simulink library "PELIIONPACK01MSEREF"  (R2014b)
settings: Solver=ode45  StartTime=0.0  StopTime=10.0  RelTol=1e-3
undefined symbols (not defined in the file): errordlg
libraries: simulink x19
settings Model: Creator=NMN6KOR  LastModifiedBy=hj82sh

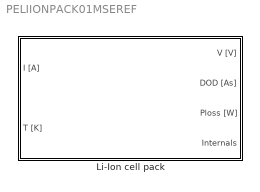
== system PELIIONPACK01MSEREF ==
  Li-Ion cell pack : Subsystem  Tag=PELIIONPACK01MSEREF  mask(PELIIONPACK01MSEREF){NumCell=1, DODtab=[0 : 23.5176 : 4680 4680], Ttab=[250 261 272 283 294 305 316 327 338 350], Vocvtab=|, Rhf=35e-3, Csn=0.01, Rct=40e-3, Cdl=700, rho=0.5, I0=0.5, T0=1.4e3, D_Rhf=[1], D_Rct=[1], D_ocv=[1], DODinit=0, VRhfinit=0, Vdlinit=0}
      mask Vocvtab=|
      | repmat( [4.10 4.09 4.09 4.08 4.08 4.08 4.08 4.07 4.07 4.07, ...
      |  4.07 4.06 4.06 4.06 4.06 4.06 4.05 4.05 4.05 4.05, ...
      |  4.05 4.04 4.04 4.04 4.04 4.04 4.03 4.03 4.03 4.02, ...
      |  4.02 4.02 4.01 4.01 4.01 4.00 4.00 3.99 3.99 3.99, ...
      |  3.98 3.98 3.98 3.97 3.97 3.96 3.96 3.96 3.95 3.95, ...
      |  3.95 3.94 3.94 3.94 3.94 3.93 3.93 3.93 3.92 3.92, ...
      |  3.92 3.92 3.91 3.91 3.91 3.90 3.90 3.90 3.89 3.89, ...
      |  3.88 3.88 3.87 3.87 3.86 3.86 3.86 3.86 3.85 3.85, ...
      |  3.85 3.84 3.84 3.84 3.84 3.83 3.83 3.83 3.82 3.82, ...
      |  3.82 3.81 3.81 3.81 3.80 3.80 3.80 3.79 3.79 3.78, ...
      |  3.78 3.78 3.77 3.77 3.76 3.76 3.75 3.75 3.74 3.74, ...
      |  3.73 3.73 3.72 3.72 3.71 3.71 3.70 3.70 3.69 3.69, ...
      |  3.68 3.68 3.67 3.67 3.67 3.66 3.66 3.65 3.65 3.65, ...
      |  3.64 3.64 3.63 3.63 3.63 3.62 3.62 3.62 3.61 3.61, ...
      |  3.60 3.60 3.60 3.59 3.59 3.58 3.58 3.58 3.57 3.57, ...
      |  3.56 3.56 3.55 3.55 3.54 3.54 3.53 3.53 3.52 3.51, ...
      |  3.51 3.50 3.50 3.49 3.48 3.48 3.47 3.47 3.46 3.45, ...
      |  3.45 3.44 3.43 3.43 3.42 3.42 3.41 3.41 3.40 3.40, ...
      |  3.39 3.39 3.38 3.37 3.37 3.36 3.35 3.34 3.33 3.31, ...
      |  3.29 3.26 3.23 3.20 3.17 3.12 3.07 3.00 2.91 2.76]', 1, 10 )
      mask prompts: NumCell "Number of cells in series connection"; DODtab "Vocv table DOD-axis [As]"; Ttab "Vocv table T-axis [K]"; Vocvtab "Vocv table [V]"; Rhf "High frequency resistance [Ohm]"; Csn "Snubber capacitance [F]"; Rct "Charge transfer resistance [Ohm]"; Cdl "Double layer capacitance [F]"; rho "Weighting factor for current dependency [-]"; I0 "Scale factor for current dependency [A]"; T0 "Scale factor for temperature dependency [K]"; D_Rhf "Rhf deviation vector [-]"; D_Rct "Rct deviation vector [-]"; D_ocv "Vocv deviation vector [-]"; DODinit "Initial depth of discharge [As]"; VRhfinit "Initial high frequency resistor voltage [V]"; Vdlinit "Initial double layer voltage [V]"
      mask help:
      | PELIIONPACK01MSEREF - Li-Ion cell pack model
      |
      | This is a simple equivalent circuit model for a series connection of Li-Ion secondary batteries. This impedance model describes the dynamical behavior of arbitrarily many cells connected in series (a subcase of this is the model of the single Li-Ion cell).
      | The number of cells determines the dimension of the input temperature vector.
      settings: AttributesFormatString=<%<Tag>>
      mask Help: eval('show_docs_mseref_powerelectronics(''PELIIONPACK01MSEREF'')')
      mask Display:
      | image(imread('PELIIONPACK01MSEREF_icon.png'))
      | port_label('input',1,'I [A]')
      | port_label('input',2,'T [K]')
      | port_label('output',1,'V [V]')
      | port_label('output',2,'DOD [As]')
      | port_label('output',3,'Ploss [W]')
      | port_label('output',4,'Internals')

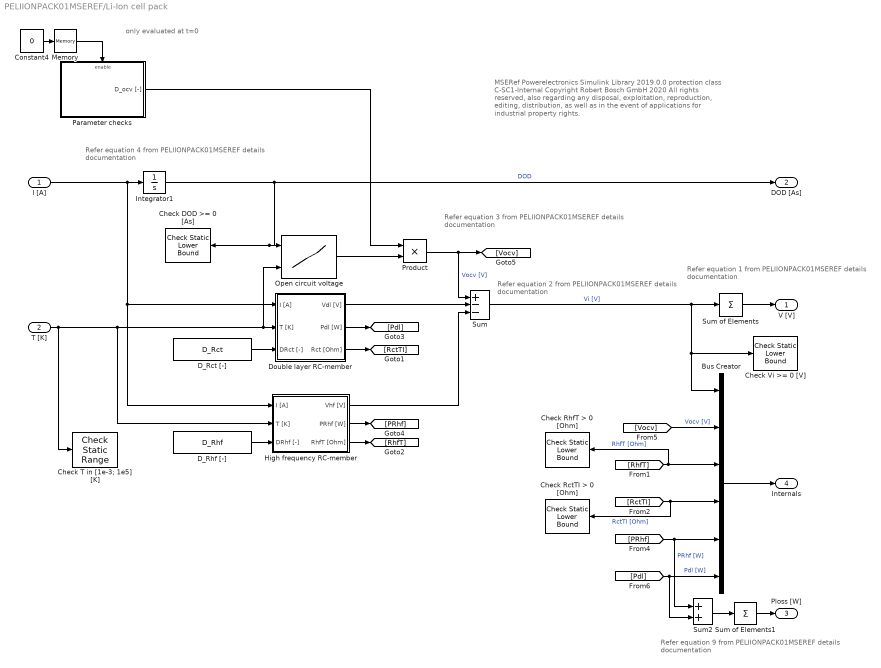
== system PELIIONPACK01MSEREF/Li-Ion cell pack ==
  note: Refer equation 9 from
      | PELIIONPACK01MSEREF details documentation
  note: Refer equation 2 from
      | PELIIONPACK01MSEREF details documentation
  note: Refer equation 4 from
      | PELIIONPACK01MSEREF details documentation
  note: only evaluated at t=0
  note: MSERef Powerelectronics Simulink Library 2019.0.0
      | protection class C-SC1-Internal
      |
      | Copyright Robert Bosch GmbH 2020
      |
      | All rights reserved, also regarding any disposal, exploitation,
      | reproduction, editing, distribution, as well as in the event of
      | applications for industrial property rights.
  note: Refer equation 1 from
      | PELIIONPACK01MSEREF details documentation
  note: Refer equation 3 from
      | PELIIONPACK01MSEREF details documentation
  I [A] : Inport
  T [K] : Inport  Port=2
  Bus Creator : BusCreator  Inputs=6
  Check DOD >= 0 [As] : simulink/Model Verification/Check Static  Lower Bound  Description=0 <= u  min=0  min_included=on  enabled=on  callback=errordlg('Output depth of discharge `DOD` has to be greater or equal to zero [As].')  stopWhenAssertionFail=on  export=off  icon=graphic
  Check RctTI > 0 [Ohm] : simulink/Model Verification/Check Static  Lower Bound  Description=0 <= u  min=0  min_included=on  enabled=on  callback=errordlg('Internal variable `RctTI` must have elements greater than zero [Ohm]. Possible reasons: Input port 3 `DeviVec`is unconnected, grounded or RhfT,i resp. RctTI,i is equal to zero.')  stopWhenAssertionFail=on  export=off  icon=graphic
  Check RhfT > 0 [Ohm] : simulink/Model Verification/Check Static  Lower Bound  Description=0 <= u  min=0  min_included=on  enabled=on  callback=errordlg('Internal variable `RhfT` must have elements greater than zero [Ohm]. Possible reasons: Input port 3 `DeviVec`is unconnected, grounded or RhfT,i resp. RctTI,i is equal to zero.')  stopWhenAssertionFail=on  export=off  icon=graphic
  Check Vi >= 0 [V] : simulink/Model Verification/Check Static  Lower Bound  Description=0 <= u  min=0  min_included=on  enabled=on  callback=errordlg('Terminal voltage `Vi` has to be greater or equal to zero [V].')  stopWhenAssertionFail=on  export=off  icon=graphic
  Check T in [1e-3; 1e5] [K] : simulink/Model Verification/Check  Static Range  Description=1e-3 <= u <= 1e5  max=1e5  max_included=on  min=1e-3  min_included=on  enabled=on  callback=errordlg('Input temperature `T` outside of range [1e-3; 1e5] [K].')  stopWhenAssertionFail=on  export=off  icon=graphic
  Constant4 : Constant  Value=0
  D_Rct [-] : Constant  Value=D_Rct
  D_Rhf [-] : Constant  Value=D_Rhf
  Double layer RC-member : Subsystem
  High frequency RC-member : Subsystem
  Integrator1 : Integrator  InitialCondition=DODinit
  Memory : Memory  X0=1
  Open circuit voltage : Lookup2D  RowIndex=DODtab  ColumnIndex=Ttab  Table=Vocvtab  LookUpMeth=Interpolation-Use End Values
  Parameter checks : Subsystem
  Product : Product
  Sum : Sum  Inputs=+--
  Sum of Elements : Sum  Inputs=+
  Sum of Elements1 : Sum  Inputs=+
  Sum2 : Sum
  V [V] : Outport
  DOD [As] : Outport  Port=2
  Ploss [W] : Outport  Port=3
  Internals : Outport  Port=4
  wires:
  Memory/1 -> Parameter checks/Enable
  Constant4/1 -> Memory/1
  Integrator1/1 -> Open circuit voltage/1, Check DOD >= 0 [As]/1, DOD [As]/1  "DOD"
  High frequency RC-member/3(RhfT [Ohm]) -> [RhfT]
  Double layer RC-member/3(Rct [Ohm]) -> [RctTI]
  Bus Creator/1 -> Internals/1
  High frequency RC-member/2(PRhf [W]) -> [PRhf]
  Double layer RC-member/2(Pdl [W]) -> [Pdl]
  T [K]/1 -> High frequency RC-member/2(T [K]), Double layer RC-member/2(T [K]), Open circuit voltage/2, Check T in [1e-3; 1e5] [K]/1
  Sum2/1 -> Sum of Elements1/1
  High frequency RC-member/1(Vhf [V]) -> Sum/3
  Double layer RC-member/1(Vdl [V]) -> Sum/2
  Open circuit voltage/1 -> Product/2
  I [A]/1 -> High frequency RC-member/1(I [A]), Double layer RC-member/1(I [A]), Integrator1/1
  [RhfT] -> Bus Creator/3, Check RhfT > 0 [Ohm]/1  "RhfT [Ohm]"
  [Vocv] -> Bus Creator/2  "Vocv [V]"
  Sum/1 -> Sum of Elements/1, Check Vi >= 0 [V]/1, Bus Creator/1  "Vi [V]"
  [RctTI] -> Check RctTI > 0 [Ohm]/1, Bus Creator/4  "RctTI [Ohm]"
  [PRhf] -> Sum2/1, Bus Creator/5  "PRhf [W]"
  [Pdl] -> Sum2/2, Bus Creator/6  "Pdl [W]"
  D_Rhf [-]/1 -> High frequency RC-member/3(DRhf [-])
  D_Rct [-]/1 -> Double layer RC-member/3(DRct [-])
  Sum of Elements/1 -> V [V]/1
  Product/1 -> Sum/1, [Vocv]  "Vocv [V]"
  Parameter checks/1(D_ocv [-]) -> Product/1
  Sum of Elements1/1 -> Ploss [W]/1

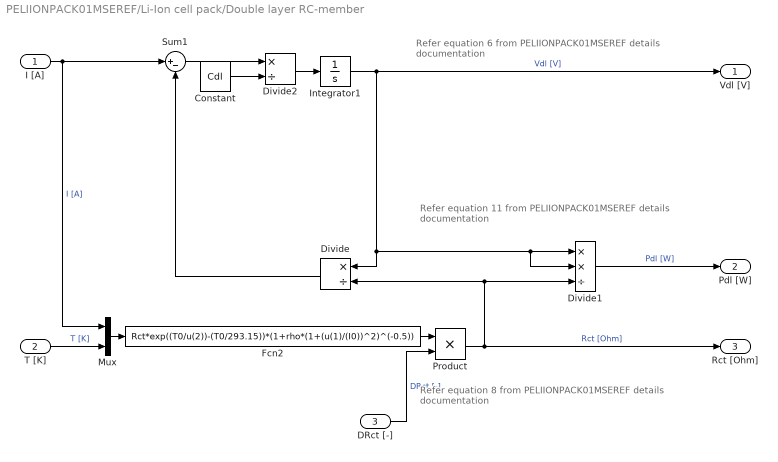
== system PELIIONPACK01MSEREF/Li-Ion cell pack/Double layer RC-member ==
  note: Refer equation 6 from
      | PELIIONPACK01MSEREF details documentation
  note: Refer equation 11 from
      | PELIIONPACK01MSEREF details documentation
  note: Refer equation 8 from
      | PELIIONPACK01MSEREF details documentation
  I [A] : Inport
  T [K] : Inport  Port=2
  DRct [-] : Inport  Port=3
  Constant : Constant  Value=Cdl
  Divide : Product  Inputs=*/
  Divide1 : Product  Inputs=**/
  Divide2 : Product  Inputs=*/
  Fcn2 : Fcn  Expr=Rct*exp((T0/u(2))-(T0/293.15))*(1+rho*(1+(u(1)/(I0))^2)^(-0.5))
  Integrator1 : Integrator  InitialCondition=Vdlinit
  Mux : Mux  Inputs=2
  Product : Product
  Sum1 : Sum  Inputs=|+-
  Vdl [V] : Outport
  Pdl [W] : Outport  Port=2
  Rct [Ohm] : Outport  Port=3
  wires:
  T [K]/1 -> Mux/2  "T [K]"
  Divide2/1 -> Integrator1/1
  Sum1/1 -> Divide2/1
  Divide1/1 -> Pdl [W]/1  "Pdl [W]"
  I [A]/1 -> Sum1/1, Mux/1  "I [A]"
  Product/1 -> Rct [Ohm]/1, Divide1/3, Divide/2  "Rct [Ohm]"
  Integrator1/1 -> Divide1/2, Divide1/1, Divide/1, Vdl [V]/1  "Vdl [V]"
  Divide/1 -> Sum1/2
  Constant/1 -> Divide2/2
  DRct [-]/1 -> Product/2  "DRct [-]"
  Mux/1 -> Fcn2/1
  Fcn2/1 -> Product/1

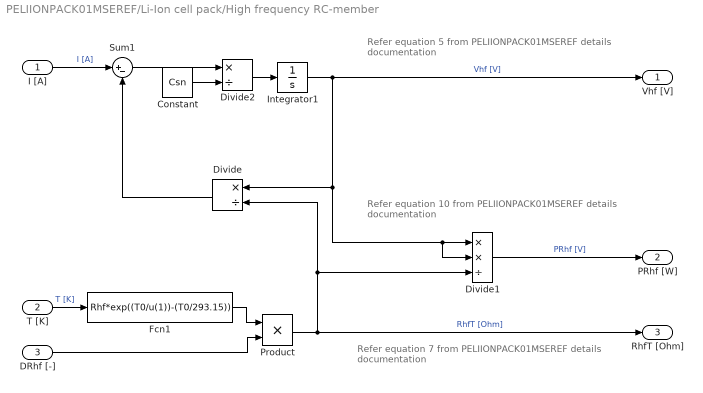
== system PELIIONPACK01MSEREF/Li-Ion cell pack/High frequency RC-member ==
  note: Refer equation 7 from
      | PELIIONPACK01MSEREF details documentation
  note: Refer equation 5 from
      | PELIIONPACK01MSEREF details documentation
  note: Refer equation 10 from
      | PELIIONPACK01MSEREF details documentation
  I [A] : Inport
  T [K] : Inport  Port=2
  DRhf [-] : Inport  Port=3
  Constant : Constant  Value=Csn
  Divide : Product  Inputs=*/
  Divide1 : Product  Inputs=**/
  Divide2 : Product  Inputs=*/
  Fcn1 : Fcn  Expr=Rhf*exp((T0/u(1))-(T0/293.15))
  Integrator1 : Integrator  InitialCondition=VRhfinit
  Product : Product
  Sum1 : Sum  Inputs=|+-
  Vhf [V] : Outport
  PRhf [W] : Outport  Port=2
  RhfT [Ohm] : Outport  Port=3
  wires:
  Divide1/1 -> PRhf [W]/1  "PRhf [V]"
  Divide2/1 -> Integrator1/1
  Divide/1 -> Sum1/2
  Product/1 -> Divide1/3, Divide/2, RhfT [Ohm]/1  "RhfT [Ohm]"
  Sum1/1 -> Divide2/1
  Integrator1/1 -> Divide1/2, Divide1/1, Divide/1, Vhf [V]/1  "Vhf [V]"
  I [A]/1 -> Sum1/1  "I [A]"
  T [K]/1 -> Fcn1/1  "T [K]"
  Constant/1 -> Divide2/2
  Fcn1/1 -> Product/1
  DRhf [-]/1 -> Product/2

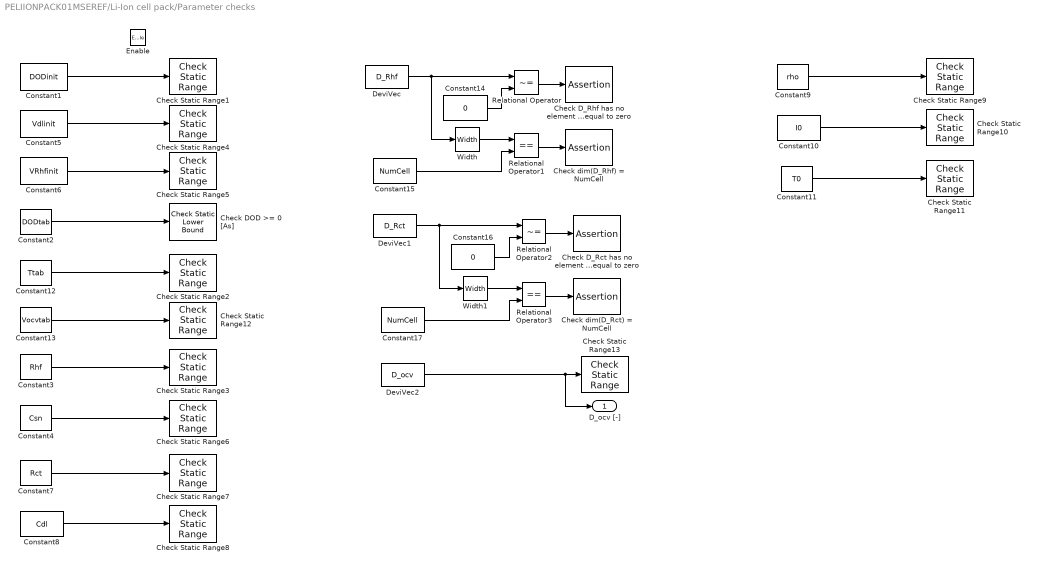
== system PELIIONPACK01MSEREF/Li-Ion cell pack/Parameter checks ==
  Enable : EnablePort  ZeroCross=off
  Check DOD >= 0 [As] : simulink/Model Verification/Check Static  Lower Bound  Description=0 <= u  min=0  min_included=on  enabled=on  callback=errordlg('Parameter Vocv table DOD-axis `DODtab` must have all elements greater or equal to zero [As].')  stopWhenAssertionFail=on  export=off  icon=graphic
  Check Static Range1 : simulink/Model Verification/Check  Static Range  Description=0 <= u <= 1e5  max=1e5  max_included=on  min=0  min_included=on  enabled=on  callback=errordlg('Parameter `Initial depth of discharge` DODinit outside boundary [0, 1e5] As.')  stopWhenAssertionFail=on  export=off  icon=graphic
  Check Static Range10 : simulink/Model Verification/Check  Static Range  Description=0 <= u <= 1e9  max=1e9  max_included=on  min=0  min_included=on  enabled=on  callback=errordlg('Parameter `Scale factor for current dependency` I0 outside boundary ]0, 1e9] A.')  stopWhenAssertionFail=on  export=off  icon=graphic
  Check Static Range11 : simulink/Model Verification/Check  Static Range  Description=0 <= u <= 1e9  max=1e9  max_included=on  min=0  min_included=on  enabled=on  callback=errordlg('Parameter `Scale factor for temperature dependency` T0 outside boundary [0, 1e9] K.')  stopWhenAssertionFail=on  export=off  icon=graphic
  Check Static Range12 : simulink/Model Verification/Check  Static Range  Description=0 <= u <= 1e9  max=1e9  max_included=on  min=0  min_included=on  enabled=on  callback=errordlg('Parameter `Vocv table` Vocvtab has elements outside boundary [0, 1e9] K.')  stopWhenAssertionFail=on  export=off  icon=graphic
  Check Static Range13 : simulink/Model Verification/Check  Static Range  Description=0 <= u <= 1e9  max=1e9  max_included=on  min=0  min_included=on  enabled=on  callback=errordlg('Parameter `Vocv deviation vector` D_ocv not in the range [0, 1e9].')  stopWhenAssertionFail=on  export=off  icon=graphic
  Check Static Range2 : simulink/Model Verification/Check  Static Range  Description=0 < u <= 1e9  max=1e9  max_included=on  min=0  min_included=off  enabled=on  callback=errordlg('Parameter `Vocv table T-axis` Ttab has elements outside boundary ]0, 1e9] K.')  stopWhenAssertionFail=on  export=off  icon=graphic
  Check Static Range3 : simulink/Model Verification/Check  Static Range  Description=0 < u <= 1e9  max=1e9  max_included=on  min=0  min_included=off  enabled=on  callback=errordlg('Parameter `High frequency resistance` Rhf outside boundary ]0, 1e9] Ohm.')  stopWhenAssertionFail=on  export=off  icon=graphic
  Check Static Range4 : simulink/Model Verification/Check  Static Range  Description=-1e9 <= u <= 1e9  max=1e9  max_included=on  min=-1e9  min_included=on  enabled=on  callback=errordlg('Parameter `Initial double layer voltage` Vdlinit outside boundary [-1e9, 1e9] V.')  stopWhenAssertionFail=on  export=off  icon=graphic
  Check Static Range5 : simulink/Model Verification/Check  Static Range  Description=-1e9 <= u <= 1e9  max=1e9  max_included=on  min=-1e9  min_included=on  enabled=on  callback=errordlg('Parameter `Initial high frequency resistor voltage` VRhfinit outside boundary [-1e9, 1e9] V.')  stopWhenAssertionFail=on  export=off  icon=graphic
  Check Static Range6 : simulink/Model Verification/Check  Static Range  Description=0 < u <= 1e9  max=1e9  max_included=on  min=0  min_included=off  enabled=on  callback=errordlg('Parameter `Snubber capacitance` Csn outside boundary ]0, 1e9] F.')  stopWhenAssertionFail=on  export=off  icon=graphic
  Check Static Range7 : simulink/Model Verification/Check  Static Range  Description=0 < u <= 1e9  max=1e9  max_included=on  min=0  min_included=off  enabled=on  callback=errordlg('Parameter `Charge transfer resistance` Rct outside boundary ]0, 1e9] Ohm.')  stopWhenAssertionFail=on  export=off  icon=graphic
  Check Static Range8 : simulink/Model Verification/Check  Static Range  Description=0 < u <= 1e9  max=1e9  max_included=on  min=0  min_included=off  enabled=on  callback=errordlg('Parameter `Double layer capacitance` Cdl outside boundary ]0, 1e9] F.')  stopWhenAssertionFail=on  export=off  icon=graphic
  Check Static Range9 : simulink/Model Verification/Check  Static Range  Description=0 <= u <= 1e9  max=1e9  max_included=on  min=0  min_included=on  enabled=on  callback=errordlg('Parameter `Weighting factor for current dependency` rho outside boundary [0, 1e9] .')  stopWhenAssertionFail=on  export=off  icon=graphic
  Check D_Rct has no element equal to zero : Assertion  AssertionFailFcn=errordlg('Parameter `Rct deviation vector` R_ct has elements equal to 0.')
  Check D_Rhf has no element equal to zero : Assertion  AssertionFailFcn=errordlg('Parameter `Rhf deviation vector` R_hf has elements equal to 0.')
  Check dim(D_Rct) = NumCell : Assertion  AssertionFailFcn=errordlg('Parameter `Rhf deviation vector` D_Rct has a dimension not equal to NumCell.')
  Check dim(D_Rhf) = NumCell : Assertion  AssertionFailFcn=errordlg('Parameter `Rhf deviation vector` D_Rhf has a dimension not equal to NumCell.')
  Constant1 : Constant  Value=DODinit
  Constant10 : Constant  Value=I0
  Constant11 : Constant  Value=T0
  Constant12 : Constant  Value=Ttab
  Constant13 : Constant  Value=Vocvtab
  Constant14 : Constant  Value=0
  Constant15 : Constant  Value=NumCell
  Constant16 : Constant  Value=0
  Constant17 : Constant  Value=NumCell
  Constant2 : Constant  Value=DODtab
  Constant3 : Constant  Value=Rhf
  Constant4 : Constant  Value=Csn
  Constant5 : Constant  Value=Vdlinit
  Constant6 : Constant  Value=VRhfinit
  Constant7 : Constant  Value=Rct
  Constant8 : Constant  Value=Cdl
  Constant9 : Constant  Value=rho
  DeviVec : Constant  Value=D_Rhf
  DeviVec1 : Constant  Value=D_Rct
  DeviVec2 : Constant  Value=D_ocv
  Relational Operator : RelationalOperator  Operator=~=  OutDataTypeStr=boolean
  Relational Operator1 : RelationalOperator  Operator===  OutDataTypeStr=boolean
  Relational Operator2 : RelationalOperator  Operator=~=  OutDataTypeStr=boolean
  Relational Operator3 : RelationalOperator  Operator===  OutDataTypeStr=boolean
  Width : Width
  Width1 : Width
  D_ocv [-] : Outport
  wires:
  Constant11/1 -> Check Static Range11/1
  Constant10/1 -> Check Static Range10/1
  Constant9/1 -> Check Static Range9/1
  Constant8/1 -> Check Static Range8/1
  Constant7/1 -> Check Static Range7/1
  Constant4/1 -> Check Static Range6/1
  Constant3/1 -> Check Static Range3/1
  Constant6/1 -> Check Static Range5/1
  Constant5/1 -> Check Static Range4/1
  Constant1/1 -> Check Static Range1/1
  Constant2/1 -> Check DOD >= 0 [As]/1
  Constant12/1 -> Check Static Range2/1
  Constant13/1 -> Check Static Range12/1
  Relational Operator/1 -> Check D_Rhf has no element equal to zero/1
  Constant14/1 -> Relational Operator/2
  DeviVec/1 -> Width/1, Relational Operator/1
  Constant15/1 -> Relational Operator1/2
  Relational Operator1/1 -> Check dim(D_Rhf) = NumCell/1
  Width/1 -> Relational Operator1/1
  Relational Operator2/1 -> Check D_Rct has no element equal to zero/1
  Constant16/1 -> Relational Operator2/2
  DeviVec1/1 -> Width1/1, Relational Operator2/1
  Constant17/1 -> Relational Operator3/2
  Relational Operator3/1 -> Check dim(D_Rct) = NumCell/1
  Width1/1 -> Relational Operator3/1
  DeviVec2/1 -> D_ocv [-]/1, Check Static Range13/1
